simulink model "mech_test"  (R2016b)
settings: Solver=ode1  StartTime=0.0  StopTime=10000  FixedStep=0.01  RelTol=1e-3
undefined symbols (not defined in the file or in its folder): DiscIntNeverNeededParam
libraries: simulink x1
settings Model: Creator=root  LastModifiedBy=liana

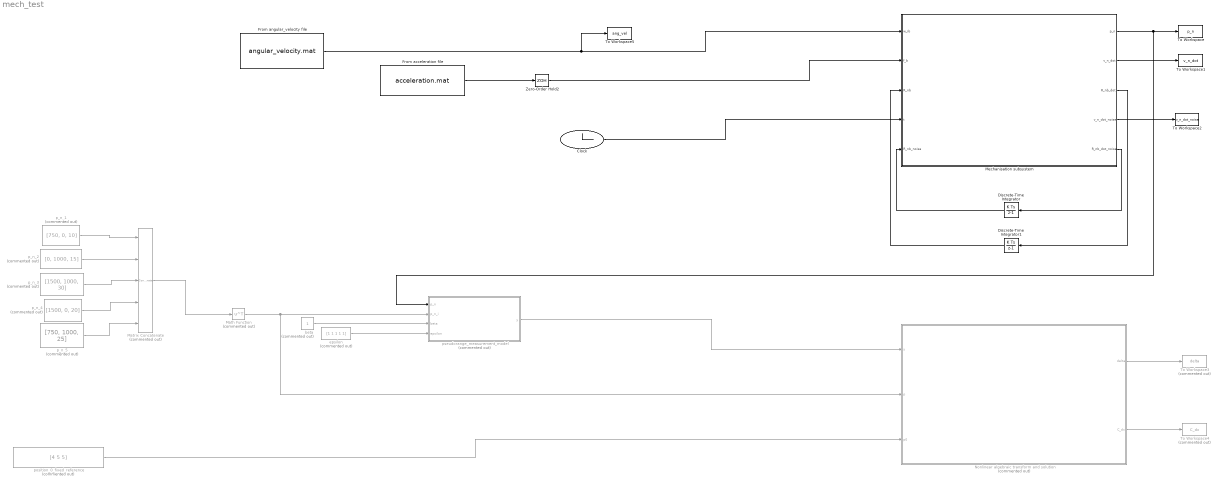
== system mech_test ==
  Clock : Clock
      settings: Decimation=50
  Discrete-Time Integrator : DiscreteIntegrator  InitialConditionSetting=State (most efficient)  SampleTime=-1  ICPrevOutput=DiscIntNeverNeededParam  ICPrevScaledInput=DiscIntNeverNeededParam
  Discrete-Time Integrator1 : DiscreteIntegrator  InitialConditionSetting=State (most efficient)  SampleTime=-1  ICPrevOutput=DiscIntNeverNeededParam  ICPrevScaledInput=DiscIntNeverNeededParam
  From acceleration file : FromFile  FileName=acceleration.mat  SampleTime=0
  From angular_velocity file : FromFile  FileName=angular_velocity.mat  SampleTime=0
  Math Function : Math  Commented=on  Operator=transpose  SaturateOnIntegerOverflow=on
  Matrix Concatenate : Concatenate  Commented=on  NumInputs=5  Mode=Multidimensional array  ConcatenateDimension=2
  Mechanisation subsystem : Subsystem
  Nonlinear algebraic transform and solution : Subsystem  Commented=on
  To Workspace : ToWorkspace  VariableName=p_n  SampleTime=-1
  To Workspace1 : ToWorkspace  VariableName=v_n_dot  SampleTime=-1
  To Workspace2 : ToWorkspace  VariableName=v_n_dot_noise  SampleTime=-1
  To Workspace3 : ToWorkspace  Commented=on  VariableName=delta  SampleTime=-1
  To Workspace4 : ToWorkspace  Commented=on  VariableName=C_dx  SampleTime=-1
  To Workspace5 : ToWorkspace  VariableName=ang_vel  SampleTime=-1
  Zero-Order Hold2 : ZeroOrderHold  SampleTime=-1
  beta : Constant  Commented=on
  epsilon : Constant  Commented=on  Value=[1 1 1 1 1]
  p_n_1 : Constant  Commented=on  Value=[750, 0, 10]
  p_n_2 : Constant  Commented=on  Value=[0, 1000, 15]
  p_n_3 : Constant  Commented=on  Value=[1500, 1000, 30]
  p_n_4 : Constant  Commented=on  Value=[1500, 0, 20]
  p_n_5 : Constant  Commented=on  Value=[750, 1000, 25]
  position_0_fixed_reference : Constant  Commented=on  Value=[4 5 5]
  pseudorange_measurement_model : MATLAB Function  Commented=on  TreatAsAtomicUnit=on
  wires:
  Clock/1 -> Mechanisation subsystem/4(t)
  From acceleration file/1 -> Zero-Order Hold2/1
  From angular_velocity file/1 -> To Workspace5/1, Mechanisation subsystem/1(w_ib)
  Zero-Order Hold2/1 -> Mechanisation subsystem/2(f_b)
  Mechanisation subsystem/5(R_nb_dot_noise) -> Discrete-Time Integrator/1
  Discrete-Time Integrator/1 -> Mechanisation subsystem/5(R_nb_noise)
  Mechanisation subsystem/3(R_nb_dot) -> Discrete-Time Integrator1/1
  Discrete-Time Integrator1/1 -> Mechanisation subsystem/3(R_nb)
  Mechanisation subsystem/2(v_n_dot) -> To Workspace1/1
  Mechanisation subsystem/4(v_n_dot_noise) -> To Workspace2/1
  pseudorange_measurement_model/1(y) -> Nonlinear algebraic transform and solution/1(y)
  beta/1 -> pseudorange_measurement_model/3(beta)
  epsilon/1 -> pseudorange_measurement_model/4(epsilon)
  Matrix Concatenate/1 -> Math Function/1
  Mechanisation subsystem/1(p_n) -> pseudorange_measurement_model/1(p_n), To Workspace/1
  p_n_5/1 -> Matrix Concatenate/5
  p_n_4/1 -> Matrix Concatenate/4
  p_n_3/1 -> Matrix Concatenate/3
  p_n_2/1 -> Matrix Concatenate/2
  p_n_1/1 -> Matrix Concatenate/1
  Math Function/1 -> Nonlinear algebraic transform and solution/2(p), pseudorange_measurement_model/2(p_n_i)
  position_0_fixed_reference/1 -> Nonlinear algebraic transform and solution/3(p0)
  Nonlinear algebraic transform and solution/1(delta) -> To Workspace3/1
  Nonlinear algebraic transform and solution/2(C_dx) -> To Workspace4/1

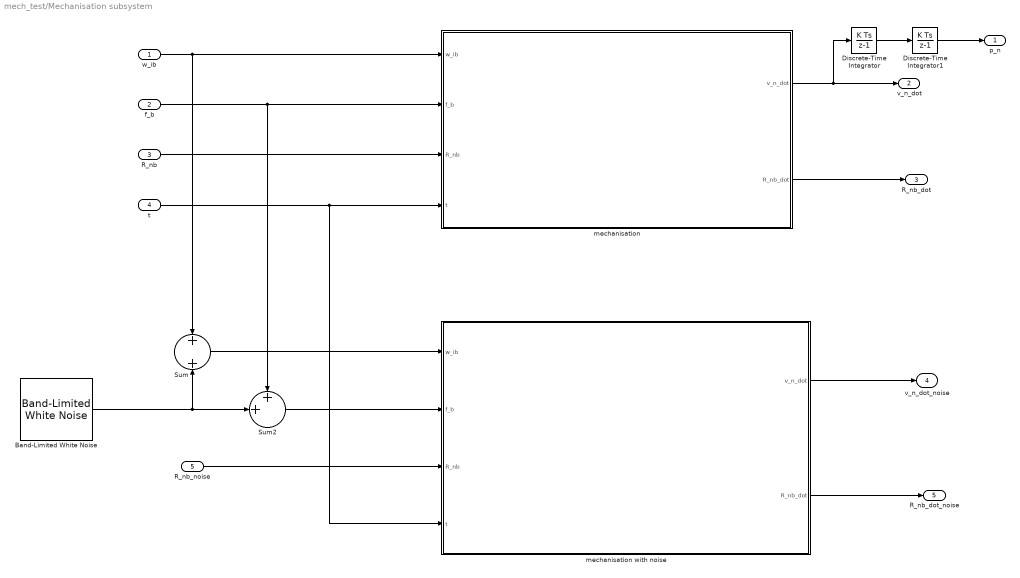
== system mech_test/Mechanisation subsystem ==
  w_ib : Inport
  f_b : Inport  Port=2
  R_nb : Inport  Port=3
  t : Inport  Port=4
  R_nb_noise : Inport  Port=5
  Band-Limited White Noise : simulink/Sources/Band-Limited White Noise  Cov=[100 100 100]'  Ts=0.1  seed=[23341]  VectorParams1D=off
  Discrete-Time Integrator : DiscreteIntegrator  InitialConditionSetting=State (most efficient)  SampleTime=-1  ICPrevOutput=DiscIntNeverNeededParam  ICPrevScaledInput=DiscIntNeverNeededParam
  Discrete-Time Integrator1 : DiscreteIntegrator  InitialConditionSetting=State (most efficient)  SampleTime=-1  ICPrevOutput=DiscIntNeverNeededParam  ICPrevScaledInput=DiscIntNeverNeededParam
  Sum : Sum  Inputs=+|+
  Sum2 : Sum  Inputs=++|
  mechanisation : MATLAB Function  TreatAsAtomicUnit=on
  mechanisation with noise : MATLAB Function  TreatAsAtomicUnit=on
  p_n : Outport
  v_n_dot : Outport  Port=2
  R_nb_dot : Outport  Port=3
  v_n_dot_noise : Outport  Port=4
  R_nb_dot_noise : Outport  Port=5
  wires:
  w_ib/1 -> mechanisation/1(w_ib), Sum/1
  t/1 -> mechanisation with noise/4(t), mechanisation/4(t)
  R_nb/1 -> mechanisation/3(R_nb)
  f_b/1 -> Sum2/1, mechanisation/2(f_b)
  mechanisation/1(v_n_dot) -> Discrete-Time Integrator/1, v_n_dot/1
  mechanisation/2(R_nb_dot) -> R_nb_dot/1
  Band-Limited White Noise/1 -> Sum/2, Sum2/2
  Sum/1 -> mechanisation with noise/1(w_ib)
  Sum2/1 -> mechanisation with noise/2(f_b)
  mechanisation with noise/1(v_n_dot) -> v_n_dot_noise/1
  mechanisation with noise/2(R_nb_dot) -> R_nb_dot_noise/1
  R_nb_noise/1 -> mechanisation with noise/3(R_nb)
  Discrete-Time Integrator/1 -> Discrete-Time Integrator1/1
  Discrete-Time Integrator1/1 -> p_n/1

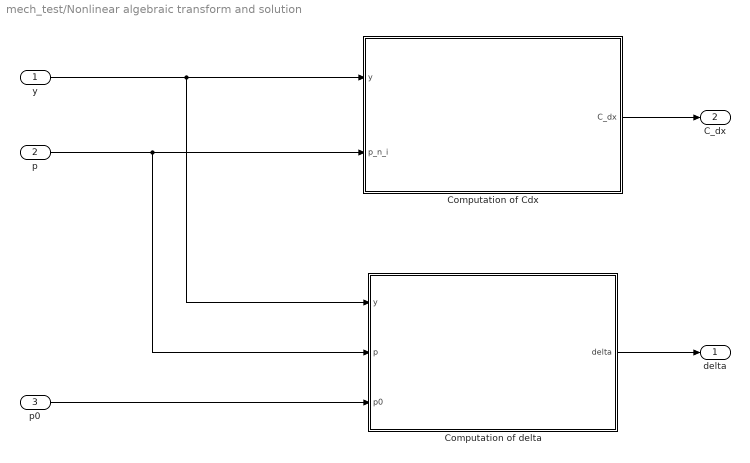
== system mech_test/Nonlinear algebraic transform and solution ==
  y : Inport
  p : Inport  Port=2
  p0 : Inport  Port=3
  Computation of Cdx : MATLAB Function  TreatAsAtomicUnit=on
  Computation of delta : MATLAB Function  TreatAsAtomicUnit=on
  delta : Outport
  C_dx : Outport  Port=2
  wires:
  y/1 -> Computation of delta/1(y), Computation of Cdx/1(y)
  p/1 -> Computation of delta/2(p), Computation of Cdx/2(p_n_i)
  p0/1 -> Computation of delta/3(p0)
  Computation of delta/1(delta) -> delta/1
  Computation of Cdx/1(C_dx) -> C_dx/1

== matlab function mech_test/Mechanisation subsystem/mechanisation ==
  data: w_ib input; f_b input; v_n_dot output; R_nb_dot output; R_nb input; t input
function [v_n_dot, R_nb_dot] = mechanisation(w_ib, f_b, R_nb, t)



g_n = [0 0 9.81]';

% w_ib = size(3,1);

if t == 0
    v_n_dot = ones(3,1);
    R_nb_dot = eye(3);
    R_nb = eye(3);
end

% mechanisation

% Skew = zeros(3,3);
% Skew(1,2) = -w_ib(3);
% Skew(2,1) = w_ib(3);
% Skew(1,3) = w_ib(2);
% Skew(3,1) = -w_ib(2);
% Skew(2,3) = -w_ib(1);
% Skew(3,2) = w_ib(1);

Skew = skew(w_ib);


%p_dot = v_n;
v_n_dot = R_nb * f_b + g_n;
R_nb_dot = R_nb * Skew;

end

== matlab function mech_test/Mechanisation subsystem/mechanisation with noise ==
  data: w_ib input; f_b input; v_n_dot output; R_nb_dot output; R_nb input; t input
function [v_n_dot, R_nb_dot] = mechanisation(w_ib, f_b, R_nb, t)



g_n = [0 0 1]';

% w_ib = size(3,1);

if t == 0
    v_n_dot = zeros(3,1);
    R_nb_dot = eye(3);
    R_nb = eye(3);
end

% mechanisation

% Skew = zeros(3,3);
% Skew(1,2) = -w_ib(3);
% Skew(2,1) = w_ib(3);
% Skew(1,3) = w_ib(2);
% Skew(3,1) = -w_ib(2);
% Skew(2,3) = -w_ib(1);
% Skew(3,2) = w_ib(1);
Skew = skew(w_ib);


%p_dot = v_n;
v_n_dot = R_nb * f_b + g_n;
R_nb_dot = R_nb * Skew;

== matlab function mech_test/Nonlinear algebraic transform and solution/Computation of Cdx ==
  data: y input; p_n_i input; C_dx output size=[4,4]
function C_dx  = C_dx_func(y,p_n_i)

    % y vector 
    % p matrix has row vectors
    %            (x,y,z) cols 
    %            m-rows are transponders number
    % all variables are in navigation frame oh yeah! baby ;)
    
    [row,col] = size(p_n_i);
    [row_,col_] = size(y);
    
    % m-measure vector
    p_m = p_n_i(row,:);
    y_m = y(row_);

    m = row; % m is transpoders number
    
    
    p_ = zeros(m-1,3); %row vector, 3 stands for x,y,z
    y_ = zeros(m-1,1);
    
    for i = 1 : 1 : m-1
    
        p_(i,:) = p_m - p_n_i(i,:);
        y_(i) = y(i) - y_m;
        
    end
    
    C_dx = [p_, y_];

end

== matlab function mech_test/Nonlinear algebraic transform and solution/Computation of delta ==
  data: y input; delta output size=4; p input; p0 input
function delta  = delta_func(y,p,p0)

    % y vector 
    % p matrix has row vectors
    %            (x,y,z) cols 
    %            m-rows are the numbers of the transponders
    % all variables are in navigation frame oh yeah! baby ;)
    % z is a col vector of scalars
    
    % we must choose p0 (a block)
    
    [row,col] = size(p);
    %[row_,col_] = size(y);
    
    p_los = zeros(row,col);
    z = zeros(row,1);
    %defining los vector
    
    for i = 1:1:row
       p_los(i,:) = p(i,:) - p0';
    end
    
    % p_los = p_los';
    
    for i = 1:1:row
        z(i)= (y(i)^2-norm(p_los(i,:))^2);
    end
    
    z = z';
    
    delta = zeros(row-1,1);
    z_m = z(end);
    
    for i = 1:1:row-1
        delta(i) =  (z(i) - z_m); %amm fenito
    end
    
    delta;

end

== matlab function mech_test/pseudorange_measurement_model ==
  data: p_n input; y output size=5; p_n_i input; beta input; epsilon input
function y = pseudorange_mea_model(p_n,p_n_i,beta,epsilon)

  %  row-vector

  y = zeros(size(p_n_i,1),1);

  for i = 1: size(p_n_i,1)

      rho = norm(p_n-p_n_i(i,:)');  % eq. 7
      
      y(i) = rho + beta + epsilon(i); % eq. 8 

  end
      
end
